simulink model "levitation"  (R2022b)
settings: Solver=ode15s  StartTime=0.0  StopTime=30  RelTol=1e-4  EnableMultiTasking=on
undefined symbols (not defined in the file): Reg_P, Reg_PI, u_bar, y1_bar, y1_ref, y2_bar
settings Model: Creator=scattolini  LastModifiedBy=Admin
settings SolverCC: AlgebraicLoopSolver=TrustRegion
settings DataIOCC: LimitDataPoints=on  SaveFormat=Array  SignalLoggingSaveFormat=ModelDataLogs  ReturnWorkspaceOutputs=off
settings OptimizationCC: ExpressionDepthLimit=2147483647  InitFltsAndDblsToZero=on  LifeSpan=inf
settings DebuggingCC: UnderspecifiedInitializationDetection=Classic  MergeDetectMultiDrivingBlocksExec=none  SolverPrmCheckMsg=warning  FcnCallInpInsideContextMsg=warning  UnconnectedInputMsg=warning  UnconnectedOutputMsg=warning  UnconnectedLineMsg=warning  StateNameClashWarn=warning  SFUnexpectedBacktrackingDiag=warning  SFNoUnconditionalDefaultTransitionDiag=warning  SFExecutionAtInitializationDiag=none  SFMachineParentedDataDiag=warning  ArithmeticOperatorsInVariantConditions=warning
settings HardwareCC: ProdBitPerPointer=32  ProdBitPerSizeT=32  ProdBitPerPtrDiffT=32  ProdLargestAtomicFloat=None  ProdIntDivRoundTo=Undefined  ProdEndianess=Unspecified  ProdWordSize=32  ProdHWDeviceType=32-bit Generic
settings ModelReferenceCC: EnableRefExpFcnMdlSchedulingChecks=on  PropagateSignalLabelsOutOfModel=off
settings SFSimCC: SimUseLocalCustomCode=off  CustomCodeUndefinedFunction=UseInterfaceOnly
settings RTWCC: RTWUseLocalCustomCode=off  DLArmComputeVersion=19.05
settings CodeAppCC: StateflowObjectComments=on
settings GRTTargetCC: TargetLangStandard=C89/C90 (ANSI)  CombineOutputUpdateFcns=off  GRTInterface=on
settings ConfigComp: CovMetricSettings=dw  CovSaveCumulativeToWorkspaceVar=on  CovSaveSingleToWorkspaceVar=on  CovExternalEMLEnable=off

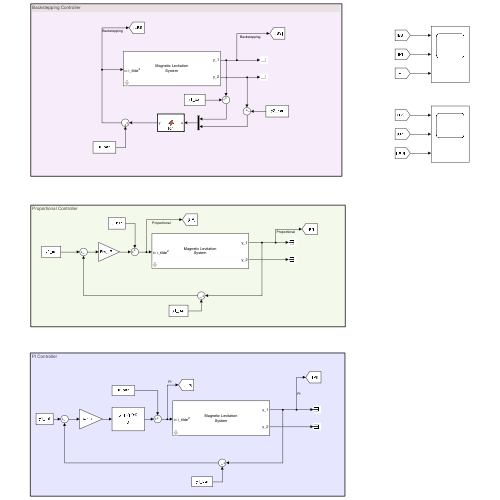
[thumbnail: Simulink's stored preview of the top-level diagram]
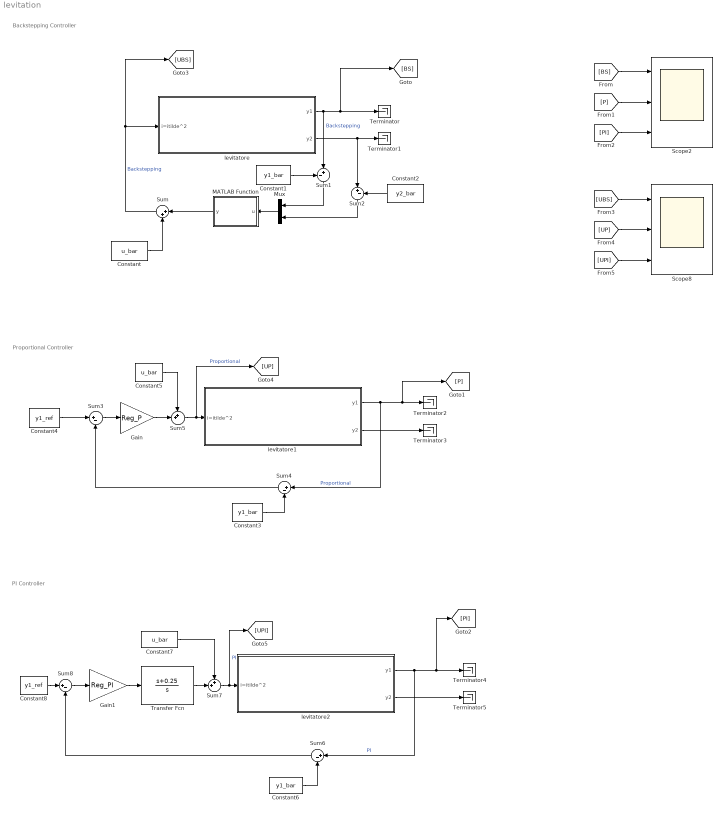
== system levitation ==
  note: Backstepping Controller
  note: Proportional Controller
  note: PI Controller
  Constant : Constant  Value=u_bar
  Constant1 : Constant  Value=y1_bar
  Constant2 : Constant  Value=y2_bar
  Constant3 : Constant  Value=y1_bar
  Constant4 : Constant  Value=y1_ref
  Constant5 : Constant  Value=u_bar
  Constant6 : Constant  Value=y1_bar
  Constant7 : Constant  Value=u_bar
  Constant8 : Constant  Value=y1_ref
  Gain : Gain  Gain=Reg_P
  Gain1 : Gain  Gain=Reg_PI
  MATLAB Function : MATLAB Function  TreatAsAtomicUnit=on
  Mux : Mux  Inputs=2
  Scope2 : Scope  NumInputPorts=3
  Scope8 : Scope  NumInputPorts=3
  Sum : Sum  Inputs=|++
  Sum1 : Sum  Inputs=-+|
  Sum{2..4,6,8} (5 alike) : Sum  Inputs=|+-
  Sum5 : Sum  Inputs=++|
  Sum7 : Sum  Inputs=++|
  Terminator{,1..5} (6 alike) : Terminator
  Transfer Fcn : TransferFcn  Numerator=[1 0.25]  Denominator=[1 0]
  levitatore : Subsystem  Description=|  mask{y1_0=1.0819, y2_0=0}
      | Magnetic Levitation System.
      | The input is the squared current. The outputs are the position (y1) and the velocity (y2).
      mask prompts: y1_0 "Initial value for y1"; y2_0 "Initial value for y2"
      mask DialogControl DescTextVar Prompt: Magnetic Levitation System. The input is the squared current. The outputs are the position (y1) and the velocity (y2).
      mask Display:
      | disp('Magnetic Levitation\nSystem');
      | port_label('input', 1, 'i= i\_tilde^2', 'texmode', 'on');
      | port_label('output', 1, 'y_1');
      | port_label('output', 2, 'y_2');
  levitatore1 : Subsystem  Description=|  mask{y1_0=1.0819, y2_0=0}
      | Magnetic Levitation System.
      | The input is the squared current. The outputs are the position (y1) and the velocity (y2).
      mask prompts: y1_0 "Initial value for y1"; y2_0 "Initial value for y2"
      mask DialogControl DescTextVar Prompt: Magnetic Levitation System. The input is the squared current. The outputs are the position (y1) and the velocity (y2).
      mask Display:
      | disp('Magnetic Levitation\nSystem');
      | port_label('input', 1, 'i= i\_tilde^2', 'texmode', 'on');
      | port_label('output', 1, 'y_1');
      | port_label('output', 2, 'y_2');
  levitatore2 : Subsystem  Description=|  mask{y1_0=1.0819, y2_0=0}
      | Magnetic Levitation System.
      | The input is the squared current. The outputs are the position (y1) and the velocity (y2).
      mask prompts: y1_0 "Initial value for y1"; y2_0 "Initial value for y2"
      mask DialogControl DescTextVar Prompt: Magnetic Levitation System. The input is the squared current. The outputs are the position (y1) and the velocity (y2).
      mask Display:
      | disp('Magnetic Levitation\nSystem');
      | port_label('input', 1, 'i= i\_tilde^2', 'texmode', 'on');
      | port_label('output', 1, 'y_1');
      | port_label('output', 2, 'y_2');
  wires:
  levitatore/1(y1) -> Sum1/2, Terminator/1, [BS]  "Backstepping"
  levitatore/2(y2) -> Terminator1/1, Sum2/1
  Mux/1 -> MATLAB Function/1(u)
  MATLAB Function/1(y) -> Sum/1
  Sum/1 -> [UBS], levitatore/1(i=itilde^2)  "Backstepping"
  Constant/1 -> Sum/2
  Constant1/1 -> Sum1/1
  Constant2/1 -> Sum2/2
  Sum1/1 -> Mux/1
  Sum2/1 -> Mux/2
  levitatore1/2(y2) -> Terminator3/1
  levitatore1/1(y1) -> Sum4/1, Terminator2/1, [P]  "Proportional"
  Gain/1 -> Sum5/2
  Sum3/1 -> Gain/1
  Sum4/1 -> Sum3/2
  Constant3/1 -> Sum4/2
  Constant4/1 -> Sum3/1
  Sum5/1 -> [UP], levitatore1/1(i=itilde^2)  "Proportional"
  Constant5/1 -> Sum5/1
  Constant7/1 -> Sum7/1
  levitatore2/2(y2) -> Terminator5/1
  Sum7/1 -> [UPI], levitatore2/1(i=itilde^2)  "PI"
  Constant6/1 -> Sum6/2
  Sum6/1 -> Sum8/2
  levitatore2/1(y1) -> Sum6/1, Terminator4/1, [PI]  "PI"
  Transfer Fcn/1 -> Sum7/2
  Constant8/1 -> Sum8/1
  Sum8/1 -> Gain1/1
  Gain1/1 -> Transfer Fcn/1
  [BS] -> Scope2/1
  [P] -> Scope2/2
  [PI] -> Scope2/3
  [UBS] -> Scope8/1
  [UP] -> Scope8/2
  [UPI] -> Scope8/3

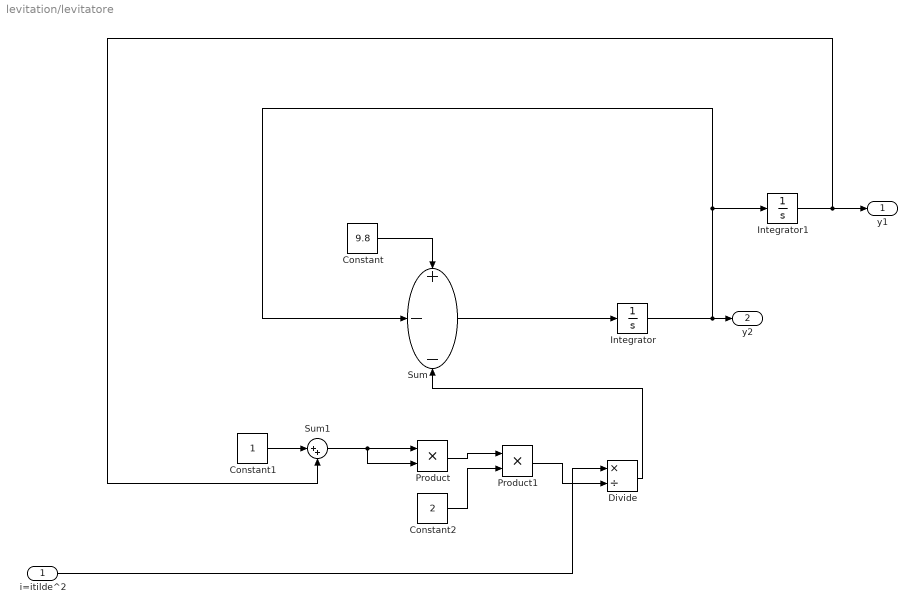
== system levitation/levitatore ==
  i=itilde^2 : Inport
  Constant : Constant  Value=9.8
  Constant1 : Constant
  Constant2 : Constant  Value=2
  Divide : Product  Inputs=*/
  Integrator : Integrator  InitialCondition=y2_0
  Integrator1 : Integrator  InitialCondition=y1_0
  Product : Product  RndMeth=Zero
  Product1 : Product  RndMeth=Zero
  Sum : Sum  Inputs=+--
  Sum1 : Sum  Inputs=|++
  y1 : Outport
  y2 : Outport  Port=2
  wires:
  Constant/1 -> Sum/1
  Constant1/1 -> Sum1/1
  Sum1/1 -> Product/1, Product/2
  Product/1 -> Product1/1
  Constant2/1 -> Product1/2
  Product1/1 -> Divide/2
  i=itilde^2/1 -> Divide/1
  Divide/1 -> Sum/3
  Sum/1 -> Integrator/1
  Integrator/1 -> Sum/2, Integrator1/1, y2/1
  Integrator1/1 -> Sum1/2, y1/1

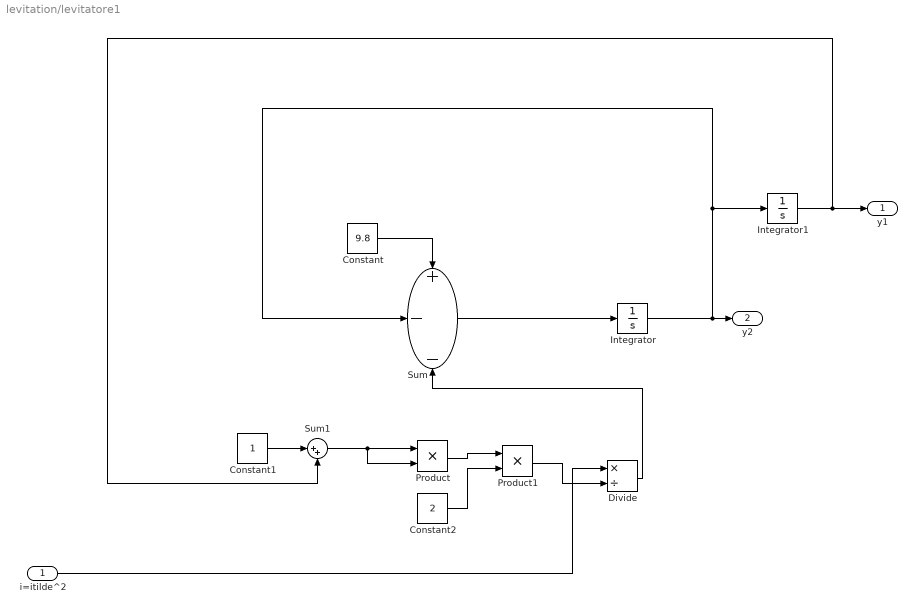
== system levitation/levitatore1 ==
  i=itilde^2 : Inport
  Constant : Constant  Value=9.8
  Constant1 : Constant
  Constant2 : Constant  Value=2
  Divide : Product  Inputs=*/
  Integrator : Integrator  InitialCondition=y2_0
  Integrator1 : Integrator  InitialCondition=y1_0
  Product : Product  RndMeth=Zero
  Product1 : Product  RndMeth=Zero
  Sum : Sum  Inputs=+--
  Sum1 : Sum  Inputs=|++
  y1 : Outport
  y2 : Outport  Port=2
  wires:
  Constant/1 -> Sum/1
  Constant1/1 -> Sum1/1
  Sum1/1 -> Product/1, Product/2
  Product/1 -> Product1/1
  Constant2/1 -> Product1/2
  Product1/1 -> Divide/2
  i=itilde^2/1 -> Divide/1
  Divide/1 -> Sum/3
  Sum/1 -> Integrator/1
  Integrator/1 -> Sum/2, Integrator1/1, y2/1
  Integrator1/1 -> Sum1/2, y1/1

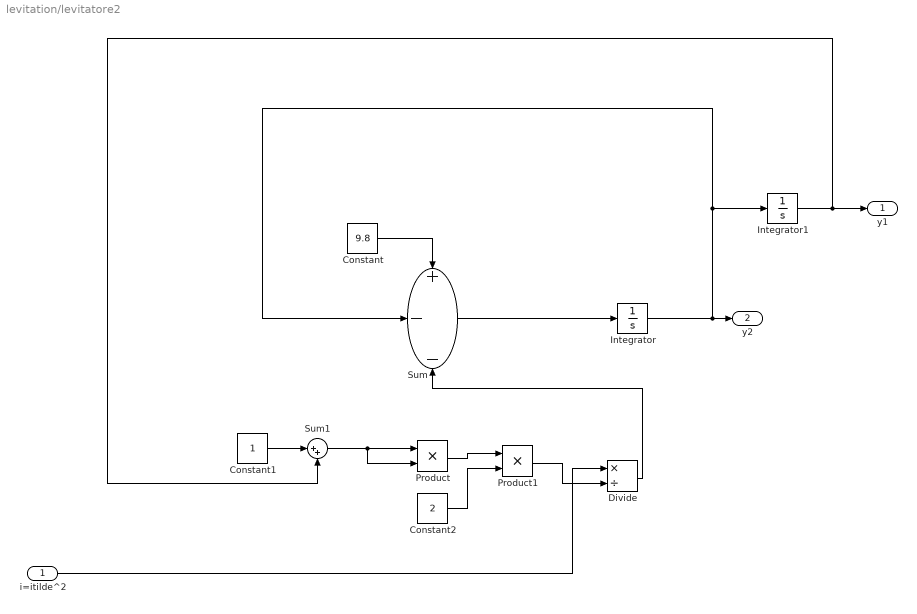
== system levitation/levitatore2 ==
  i=itilde^2 : Inport
  Constant : Constant  Value=9.8
  Constant1 : Constant
  Constant2 : Constant  Value=2
  Divide : Product  Inputs=*/
  Integrator : Integrator  InitialCondition=y2_0
  Integrator1 : Integrator  InitialCondition=y1_0
  Product : Product  RndMeth=Zero
  Product1 : Product  RndMeth=Zero
  Sum : Sum  Inputs=+--
  Sum1 : Sum  Inputs=|++
  y1 : Outport
  y2 : Outport  Port=2
  wires:
  Constant/1 -> Sum/1
  Constant1/1 -> Sum1/1
  Sum1/1 -> Product/1, Product/2
  Product/1 -> Product1/1
  Constant2/1 -> Product1/2
  Product1/1 -> Divide/2
  i=itilde^2/1 -> Divide/1
  Divide/1 -> Sum/3
  Sum/1 -> Integrator/1
  Integrator/1 -> Sum/2, Integrator1/1, y2/1
  Integrator1/1 -> Sum1/2, y1/1

== matlab function levitation/MATLAB Function ==
  data: u input; y output
function y = fcn(u)
K = 2;
g = 9.8;

y = 2 * (2 + u(1))^2 * ( (1+K) * u(1) + K * u(2) + g ) - 8*g;
